simulink model "gm_DUALportRAMinterface"  (R2024a)
settings: Solver=FixedStepDiscrete  StartTime=0.0  StopTime=2  RelTol=1e-3
undefined symbols (not defined in the file or in its folder): Ts
libraries: hdlsllib x18, simulink x1
settings Model: Creator=Simon  LastModifiedBy=Simon
settings OptimizationCC: BlockReduction=off  ConditionallyExecuteInputs=off  DefaultParameterBehavior=Inlined  InheritOutputTypeSmallerThanSingle=on
settings DebuggingCC: AlgebraicLoopMsg=error  InheritedTsInSrcMsg=none  SingleTaskRateTransMsg=error  UnconnectedInputMsg=warning  UnconnectedOutputMsg=warning  UnconnectedLineMsg=warning
settings HardwareCC: ProdBitPerPointer=32  ProdBitPerSizeT=32  ProdBitPerPtrDiffT=32  ProdLargestAtomicFloat=None  ProdIntDivRoundTo=Undefined  ProdEndianess=Unspecified  ProdWordSize=32  ProdHWDeviceType=ASIC/FPGA->ASIC/FPGA  TargetBitPerPointer=64  TargetBitPerSizeT=64  TargetBitPerPtrDiffT=64  TargetLongLongMode=on  TargetIntDivRoundTo=Zero  TargetEndianess=LittleEndian  TargetWordSize=64  TargetHWDeviceType=Custom Processor->MATLAB Host Computer  ProdEqTarget=off

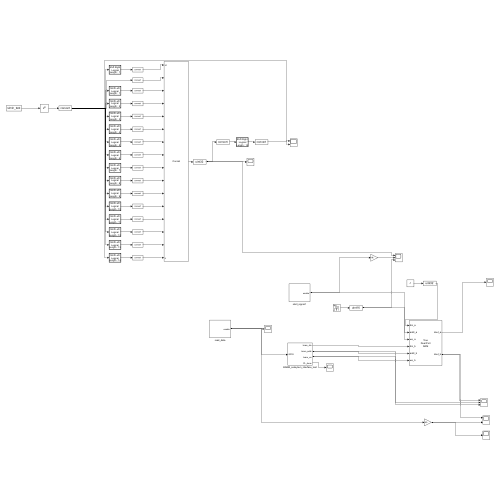
[thumbnail: Simulink's stored preview of the top-level diagram]
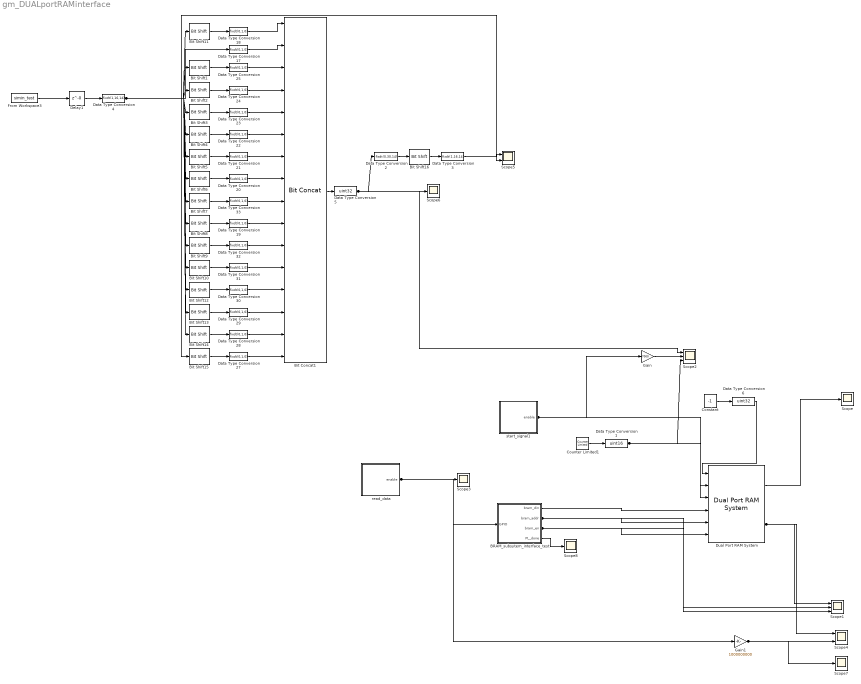
== system gm_DUALportRAMinterface ==
  BRAM_subsytem_interface_test : Subsystem
  Bit Concat1 : hdlsllib/Logic and Bit Operations/Bit Concat  numInputs=16
  Bit Shift1 : hdlsllib/Logic and Bit Operations/Bit Shift  mode=Shift Left Logical  N=1
  Bit Shift10 : hdlsllib/Logic and Bit Operations/Bit Shift  mode=Shift Left Logical  N=10
  Bit Shift11 : hdlsllib/Logic and Bit Operations/Bit Shift  mode=Shift Right Logical  N=1
  Bit Shift12 : hdlsllib/Logic and Bit Operations/Bit Shift  mode=Shift Left Logical  N=11
  Bit Shift13 : hdlsllib/Logic and Bit Operations/Bit Shift  mode=Shift Left Logical  N=12
  Bit Shift14 : hdlsllib/Logic and Bit Operations/Bit Shift  mode=Shift Left Logical  N=13
  Bit Shift15 : hdlsllib/Logic and Bit Operations/Bit Shift  mode=Shift Left Logical  N=14
  Bit Shift16 : hdlsllib/Logic and Bit Operations/Bit Shift  mode=Shift Right Logical  N=14
  Bit Shift2 : hdlsllib/Logic and Bit Operations/Bit Shift  mode=Shift Left Logical  N=2
  Bit Shift3 : hdlsllib/Logic and Bit Operations/Bit Shift  mode=Shift Left Logical  N=3
  Bit Shift4 : hdlsllib/Logic and Bit Operations/Bit Shift  mode=Shift Left Logical  N=4
  Bit Shift5 : hdlsllib/Logic and Bit Operations/Bit Shift  mode=Shift Left Logical  N=5
  Bit Shift6 : hdlsllib/Logic and Bit Operations/Bit Shift  mode=Shift Left Logical  N=6
  Bit Shift7 : hdlsllib/Logic and Bit Operations/Bit Shift  mode=Shift Left Logical  N=7
  Bit Shift8 : hdlsllib/Logic and Bit Operations/Bit Shift  mode=Shift Left Logical  N=8
  Bit Shift9 : hdlsllib/Logic and Bit Operations/Bit Shift  mode=Shift Left Logical  N=9
  Constant : Constant  Value=-1  SampleTime=-1
  Counter Limited1 : simulink/Sources/Counter Limited  uplimit=7000  tsamp=Ts
  Data Type Conversion1 : DataTypeConversion  OutDataTypeStr=uint16  SaturateOnIntegerOverflow=off  RndMeth=Floor
  Data Type Conversion{17..25,27..33} (16 alike) : DataTypeConversion  OutDataTypeStr=fixdt(0,1,0)  SaturateOnIntegerOverflow=off  RndMeth=Floor
  Data Type Conversion2 : DataTypeConversion  OutDataTypeStr=fixdt(0,30,14)  SaturateOnIntegerOverflow=off  RndMeth=Floor
  Data Type Conversion3 : DataTypeConversion  OutDataTypeStr=fixdt(1,16,14)  SaturateOnIntegerOverflow=off  RndMeth=Floor
  Data Type Conversion4 : DataTypeConversion  OutDataTypeStr=fixdt(1,16,14)  SaturateOnIntegerOverflow=off  RndMeth=Floor
  Data Type Conversion5 : DataTypeConversion  OutDataTypeStr=uint32  SaturateOnIntegerOverflow=off  RndMeth=Floor
  Data Type Conversion6 : DataTypeConversion  OutDataTypeStr=uint32  SaturateOnIntegerOverflow=off  RndMeth=Floor
  Delay1 : Delay  DelayLength=0  InitialCondition=0  SampleTime=Ts
  Dual Port RAM System : hdlsllib/HDL RAMs/Dual Port RAM System  RAMType=True dual port  AsyncRead=off  WriteOutputValue=New data  RAMInitialValue=0  allowBusInputs=off  WritesHaveOutput=on  NumReads=0  NumWrites=1  SimulateUsing=Code generation
  From Workspace3 : FromWorkspace  VariableName=simin_test  SampleTime=Ts
  Gain : Gain  Gain=7000
  Gain1 : Gain  Gain=1000000000
  Scope{,3,6..8} (5 alike) : Scope
  Scope1 : Scope  NumInputPorts=3
  Scope2 : Scope  NumInputPorts=3
  Scope4 : Scope  NumInputPorts=2
  Scope5 : Scope  NumInputPorts=2
  read_data : Subsystem
  start_signal1 : Subsystem
  wires:
  BRAM_subsytem_interface_test/4(PL_done) -> Scope8/1
  Gain1/1 -> Scope4/2, Scope7/1
  Data Type Conversion6/1 -> Dual Port RAM System/1
  Constant/1 -> Data Type Conversion6/1
  read_data/1(enable) -> BRAM_subsytem_interface_test/1(GPIO), Gain1/1, Scope3/1
  Bit Shift5/1 -> Data Type Conversion21/1
  Data Type Conversion27/1 -> Bit Concat1/16
  Data Type Conversion23/1 -> Bit Concat1/5
  Bit Shift4/1 -> Data Type Conversion22/1
  Data Type Conversion18/1 -> Bit Concat1/1
  Data Type Conversion29/1 -> Bit Concat1/14
  Bit Shift11/1 -> Data Type Conversion18/1
  Data Type Conversion25/1 -> Bit Concat1/3
  Delay1/1 -> Data Type Conversion4/1
  Data Type Conversion32/1 -> Bit Concat1/11
  Data Type Conversion24/1 -> Bit Concat1/4
  Data Type Conversion4/1 -> Bit Shift11/1, Data Type Conversion17/1, Bit Shift1/1, Bit Shift2/1, Bit Shift14/1, Bit Shift15/1, Bit Shift13/1, Bit Shift12/1, Bit Shift10/1, Bit Shift9/1, Bit Shift8/1, Bit Shift7/1, Bit Shift6/1, Bit Shift5/1, Bit Shift4/1, Bit Shift3/1, Scope5/2
  Data Type Conversion28/1 -> Bit Concat1/15
  Bit Shift15/1 -> Data Type Conversion27/1
  Data Type Conversion17/1 -> Bit Concat1/2
  Data Type Conversion21/1 -> Bit Concat1/7
  Data Type Conversion33/1 -> Bit Concat1/9
  Bit Shift9/1 -> Data Type Conversion32/1
  Bit Shift6/1 -> Data Type Conversion20/1
  Bit Shift14/1 -> Data Type Conversion28/1
  Data Type Conversion5/1 -> Data Type Conversion2/1, Scope6/1, Scope2/1
  Bit Shift7/1 -> Data Type Conversion33/1
  Bit Shift3/1 -> Data Type Conversion23/1
  From Workspace3/1 -> Delay1/1
  Data Type Conversion22/1 -> Bit Concat1/6
  Bit Concat1/1 -> Data Type Conversion5/1
  Bit Shift13/1 -> Data Type Conversion29/1
  Bit Shift12/1 -> Data Type Conversion30/1
  Bit Shift8/1 -> Data Type Conversion19/1
  Bit Shift10/1 -> Data Type Conversion31/1
  Data Type Conversion2/1 -> Bit Shift16/1
  Data Type Conversion31/1 -> Bit Concat1/12
  Data Type Conversion30/1 -> Bit Concat1/13
  Data Type Conversion20/1 -> Bit Concat1/8
  Data Type Conversion19/1 -> Bit Concat1/10
  Bit Shift2/1 -> Data Type Conversion24/1
  Bit Shift1/1 -> Data Type Conversion25/1
  Bit Shift16/1 -> Data Type Conversion3/1
  Data Type Conversion3/1 -> Scope5/1
  Gain/1 -> Scope2/2
  BRAM_subsytem_interface_test/3(bram_en) -> Dual Port RAM System/6, Scope1/3
  BRAM_subsytem_interface_test/2(bram_addr) -> Dual Port RAM System/5, Scope1/2
  BRAM_subsytem_interface_test/1(bram_din) -> Dual Port RAM System/4
  start_signal1/1(enable) -> Gain/1, Dual Port RAM System/3
  Data Type Conversion1/1 -> Dual Port RAM System/2, Scope2/3
  Counter Limited1/1 -> Data Type Conversion1/1
  Dual Port RAM System/2 -> Scope1/1, Scope4/1
  Dual Port RAM System/1 -> Scope/1

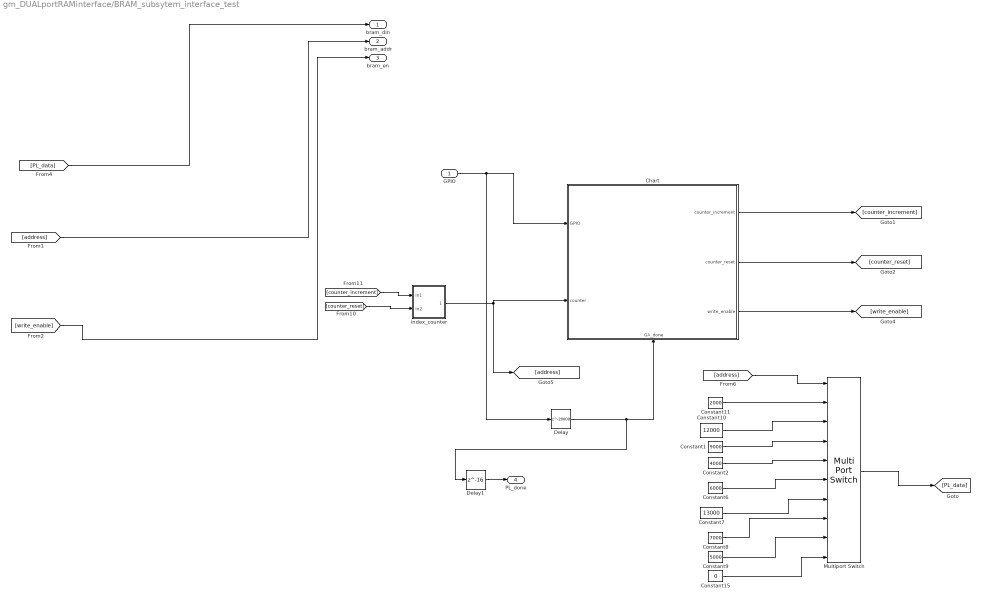
== system gm_DUALportRAMinterface/BRAM_subsytem_interface_test ==
  GPIO : Inport
  Chart : Stateflow chart  TreatAsAtomicUnit=on
      settings: PortSchema="{\"entries\":[{\"content\":{\"sides\":[{\"content\":{\"connectorIds\":[\"In2\",\"In3\"]},\"type\":\"ConnectorPlacement.EquallySpacedRectSide\",\"uuid\":\"f3ce331f-c708-4668-a9cb-fb327ea74ab5\"},{\"content\":{\"connectorIds\":[\"Out1\",\"Out2\",\"Out3\"],\"side\":\"RIGHT\"},\"type\":\"ConnectorPlacement.EquallySpacedRectSide\",\"uuid\":\"3766927a-abff-497d-9544-2098881ba174\"},{\"content\":{\"side\":\"TOP\"},\"type\":\"ConnectorPlacement.EquallySpacedRectSide\",\"uuid\":\"ebfe3d64-ee7d-4953-a6ba-e7e40988decf\"},{\"content\":{\"connectorIds\":[\"In1\"],\"side\":\"BOTTOM\"},\"type\":\"ConnectorPlacement.EquallySpacedRectSide\",\"uuid\":\"f39ceaf8-4df7-4e40-9de5-da7597831fb4\"}]},\"type\":\"ConnectorPlacement.EquallySpacedConnector\",\"uuid\":\"89f60450-5933-42bb-b72b-5f8ec55483e0\"}],\"packageUris\":[\"http://schema.mathworks.com/mf0/Connector/R2020b\"],\"version\":\"1.0\"}"
  Constant1 : Constant  Value=9000  OutDataTypeStr=uint32  SampleTime=Ts
  Constant10 : Constant  Value=12000  OutDataTypeStr=uint32  SampleTime=Ts
  Constant11 : Constant  Value=2000  OutDataTypeStr=uint32  SampleTime=Ts
  Constant15 : Constant  Value=0  OutDataTypeStr=uint32  SampleTime=Ts
  Constant2 : Constant  Value=4000  OutDataTypeStr=uint32  SampleTime=Ts
  Constant6 : Constant  Value=6000  OutDataTypeStr=uint32  SampleTime=Ts
  Constant7 : Constant  Value=13000  OutDataTypeStr=uint32  SampleTime=Ts
  Constant8 : Constant  Value=7000  OutDataTypeStr=uint32  SampleTime=Ts
  Constant9 : Constant  Value=5000  OutDataTypeStr=uint32  SampleTime=Ts
  Delay : Delay  DelayLength=20000  InitialCondition=0
  Delay1 : Delay  DelayLength=16  InitialCondition=0  SampleTime=Ts
  Multiport Switch : MultiPortSwitch  DataPortOrder=Specify indices  Inputs=8  DataPortIndices={0,1,2,3,4,5,6,7}  DataPortForDefault=Additional data port  DiagnosticForDefault=None  SaturateOnIntegerOverflow=off  InputSameDT=off
  index_counter : Subsystem
  bram_din : Outport
  bram_addr : Outport  Port=2
  bram_en : Outport  Port=3
  PL_done : Outport  Port=4
  wires:
  Delay1/1 -> PL_done/1
  Delay/1 -> Chart/1(GA_done), Delay1/1
  [write_enable] -> bram_en/1
  Constant6/1 -> Multiport Switch/6
  [PL_data] -> bram_din/1
  Constant8/1 -> Multiport Switch/8
  Constant9/1 -> Multiport Switch/9
  Chart/1(counter_increment) -> [counter_increment]
  Chart/2(counter_reset) -> [counter_reset]
  Constant10/1 -> Multiport Switch/3
  GPIO/1 -> Chart/2(GPIO), Delay/1
  Constant7/1 -> Multiport Switch/7
  Chart/3(write_enable) -> [write_enable]
  [address] -> Multiport Switch/1
  Constant11/1 -> Multiport Switch/2
  Constant15/1 -> Multiport Switch/10
  [counter_increment] -> index_counter/1(In1)
  [address] -> bram_addr/1
  Constant2/1 -> Multiport Switch/5
  Constant1/1 -> Multiport Switch/4
  index_counter/1(index_counter) -> [address], Chart/3(counter)
  [counter_reset] -> index_counter/2(In2)
  Multiport Switch/1 -> [PL_data]

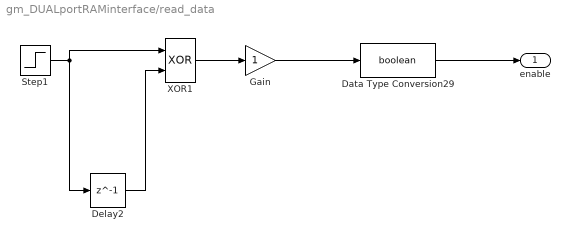
== system gm_DUALportRAMinterface/read_data ==
  Data Type Conversion29 : DataTypeConversion  OutDataTypeStr=boolean  SaturateOnIntegerOverflow=off  RndMeth=Floor
  Delay2 : Delay  DelayLength=1  InitialCondition=0  SampleTime=Ts
  Gain : Gain
  Step1 : Step  Time=Ts*7000  SampleTime=Ts
  XOR1 : Logic  Operator=XOR  IconShape=distinctive  AllPortsSameDT=off  OutDataTypeStr=boolean
  enable : Outport
  wires:
  Data Type Conversion29/1 -> enable/1
  Gain/1 -> Data Type Conversion29/1
  Delay2/1 -> XOR1/2
  Step1/1 -> XOR1/1, Delay2/1
  XOR1/1 -> Gain/1

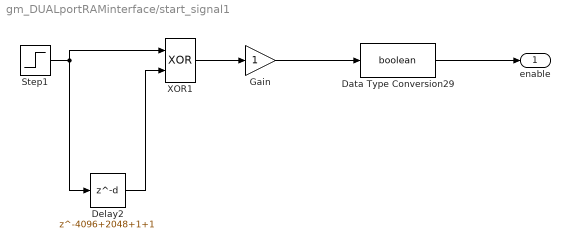
== system gm_DUALportRAMinterface/start_signal1 ==
  Data Type Conversion29 : DataTypeConversion  OutDataTypeStr=boolean  SaturateOnIntegerOverflow=off  RndMeth=Floor
  Delay2 : Delay  DelayLength=4096+2048+1+1  InitialCondition=0  SampleTime=Ts
  Gain : Gain
  Step1 : Step  Time=Ts*0  SampleTime=Ts
  XOR1 : Logic  Operator=XOR  IconShape=distinctive  AllPortsSameDT=off  OutDataTypeStr=boolean
  enable : Outport
  wires:
  XOR1/1 -> Gain/1
  Step1/1 -> Delay2/1, XOR1/1
  Delay2/1 -> XOR1/2
  Gain/1 -> Data Type Conversion29/1
  Data Type Conversion29/1 -> enable/1

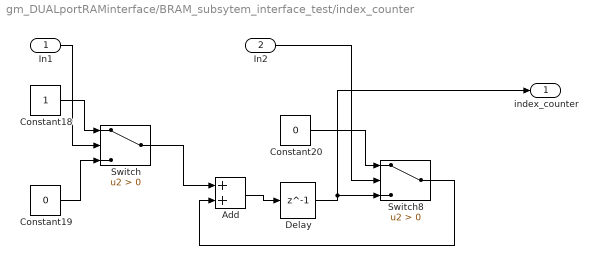
== system gm_DUALportRAMinterface/BRAM_subsytem_interface_test/index_counter ==
  In1 : Inport
  In2 : Inport  Port=2
  Add : Sum  OutDataTypeStr=Inherit: Same as first input
  Constant18 : Constant  OutDataTypeStr=fixdt(0,16,0)  SampleTime=Ts
  Constant19 : Constant  Value=0  OutDataTypeStr=fixdt(0,16,0)  SampleTime=Ts
  Constant20 : Constant  Value=0  OutDataTypeStr=uint16  SampleTime=Ts
  Delay : Delay  DelayLength=1  InitialCondition=0  SampleTime=Ts
  Switch : Switch  Criteria=u2 > Threshold  SaturateOnIntegerOverflow=off  InputSameDT=off  OutDataTypeStr=Inherit: Same as first input
  Switch8 : Switch  Criteria=u2 > Threshold  SaturateOnIntegerOverflow=off  InputSameDT=off  OutDataTypeStr=Inherit: Same as first input
  index_counter : Outport
  wires:
  In1/1 -> Switch/2
  Constant18/1 -> Switch/1
  Constant20/1 -> Switch8/1
  Add/1 -> Delay/1
  In2/1 -> Switch8/2
  Delay/1 -> Switch8/3, index_counter/1
  Switch/1 -> Add/1
  Switch8/1 -> Add/2
  Constant19/1 -> Switch/3

== stateflow chart gm_DUALportRAMinterface/BRAM_subsytem_interface_test/Chart ==
  settings: executeAtInitialization=1
  state initial_wait_state
    entry:
    counter_increment = false;
    counter_reset = true;
    write_enable = false;
  state PL_read_data
    entry:
    counter_increment = true;
    counter_reset = false;
    write_enable = false;
  state wait_for_GA_done
    entry:
    counter_increment = false;
    counter_reset = true;
    write_enable = false;
  state reset_state
    entry:
    counter_increment = false;
    counter_reset = true;
    write_enable = false;
  state PL_write_data_back
    entry:
    counter_increment = true;
    counter_reset = false;
    write_enable = true;
  (default) -> initial_wait_state
  initial_wait_state -> PL_read_data : [GPIO == 1]
  reset_state -> initial_wait_state
  PL_read_data -> wait_for_GA_done : [counter == 4096+2048+1]
  wait_for_GA_done -> PL_write_data_back : [GA_done == 1]
  PL_write_data_back -> reset_state : [counter == 8]
  data: GA_done input boolean; GPIO input; counter input; counter_increment output boolean; counter_reset output boolean; write_enable output boolean
